simulink model "StopForInstabilityObserverSpeed"  (R2016b)
settings: configuration reference "WheelSimConfiguration2016" (kept outside this file)
libraries: simulink x1
settings Model: Creator=At  LastModifiedBy=ateay
settings ConfigSetRef: SourceLocation=Base Workspace

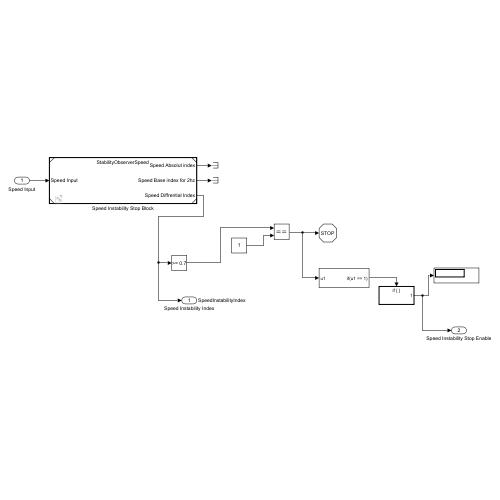
[thumbnail: Simulink's stored preview of the top-level diagram]
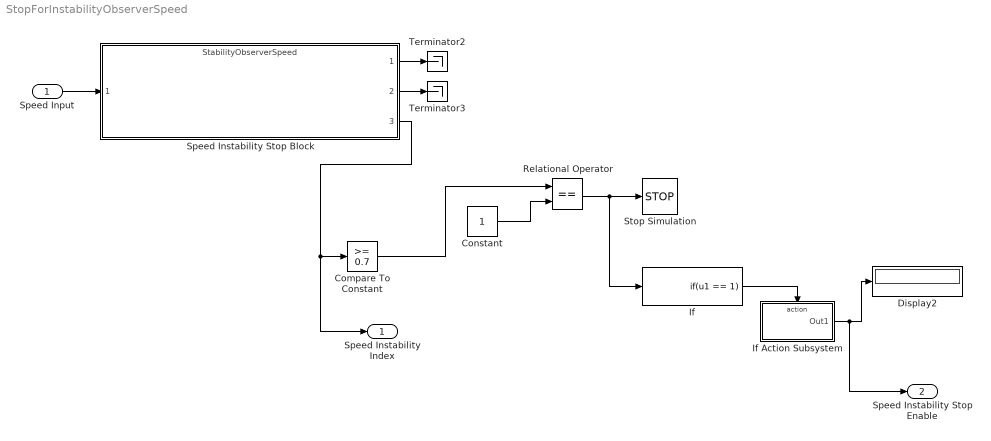
== system StopForInstabilityObserverSpeed ==
  Speed Input : Inport
  Compare To Constant : simulink/Logic and Bit Operations/Compare To Constant  relop=>=  const=0.7  OutDataTypeStr=boolean
  Constant : Constant
  Display2 : Display
  If : If  IfExpression=u1 == 1  ShowElse=off
  If Action Subsystem : Subsystem  TreatAsAtomicUnit=on
  Relational Operator : RelationalOperator  Operator===  OutDataTypeStr=boolean  RndMeth=Simplest
  Speed Instability Stop Block : ModelReference  ModelNameDialog=StabilityObserverSpeed.slx  SimulationMode=Normal  ModelReferenceVersion=1.23
  Stop Simulation : Stop
  Terminator2 : Terminator
  Terminator3 : Terminator
  Speed Instability Index : Outport  SignalName=SpeedInstabilityIndex
  Speed Instability Stop Enable : Outport  Port=2
  wires:
  Speed Instability Stop Block/3 -> Speed Instability Index/1, Compare To Constant/1
  Compare To Constant/1 -> Relational Operator/1
  Constant/1 -> Relational Operator/2
  Relational Operator/1 -> If/1, Stop Simulation/1
  If/1 -> If Action Subsystem/Action
  If Action Subsystem/1(Out1) -> Speed Instability Stop Enable/1, Display2/1
  Speed Input/1 -> Speed Instability Stop Block/1
  Speed Instability Stop Block/1 -> Terminator2/1
  Speed Instability Stop Block/2 -> Terminator3/1

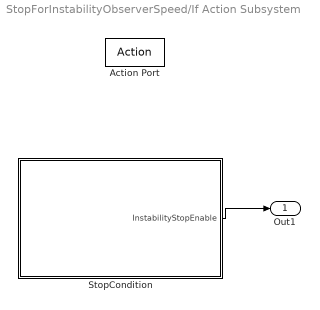
== system StopForInstabilityObserverSpeed/If Action Subsystem ==
  Action Port : ActionPort
  StopCondition : MATLAB Function  TreatAsAtomicUnit=on
  Out1 : Outport
  wires:
  StopCondition/1(InstabilityStopEnable) -> Out1/1

== matlab function StopForInstabilityObserverSpeed/If Action Subsystem/StopCondition ==
  data: InstabilityStopEnable output
function InstabilityStopEnable   = stopcondition(  )

%% This function calculates the wheel acceleration based on the simple dynamic model of propelling in a straight line


    
InstabilityStopEnable=1;
